simulink model "LCK_0112"  (R2018b)
settings: Solver=FixedStepDiscrete  StartTime=0.0  StopTime=inf  FixedStep=0.01  RelTol=1e-3
PostLoadFcn:
  | if any(exist('dsrtsu_mdlpostloadfcn', 'file') ~= 0), dsrtsu_mdlpostloadfcn('Execute', bdroot); end
values from neighbouring files (symbols this model uses):
  C_DEG2RAD = 0.0175    [LCK_Macro.sldd]
  C_KPH2MPS = 0.2778    [LCK_Macro.sldd]
  C_NEARZERO = 0.0001    [LCK_Macro.sldd]
  C_ONE = 1.0    [LCK_Macro.sldd]
  C_RAD2DEG = 57.2958    [LCK_Macro.sldd]
  C_ZERO = 0.0    [LCK_Macro.sldd]
  k_accel_pedal_pos_per_speed_x : value not decoded    [LCK_LogicPara.sldd]
  k_accel_pedal_pos_per_speed_z : value not decoded    [LCK_LogicPara.sldd]
  k_brake_suprress_hold = 1000.0    [LCK_LogicPara.sldd]
  k_driver_appl_torque_filt = 50.0    [LCK_LogicPara.sldd]
  k_driver_suppression_hold_time = 3000.0    [LCK_LogicPara.sldd]
  k_hands_on_wheel_hold_msec = 500.0    [LCK_LogicPara.sldd]
  k_hands_on_wheel_torque_hi = 0.2    [LCK_LogicPara.sldd]
  k_hands_on_wheel_torque_lo = 0.15    [LCK_LogicPara.sldd]
  k_handsoff_delay_cycles = 50.0    [LCK_LogicPara.sldd]
  k_handsoff_torq_Lo_CR = 0.3    [LCK_LogicPara.sldd]
  k_handson_delay_cycles = 5.0    [LCK_LogicPara.sldd]
  k_HighAccel_suppress_hold = 3000.0    [LCK_LogicPara.sldd]
  k_HLR_suprress_hold = 3000.0    [LCK_LogicPara.sldd]
  k_hs_StrAng_CR_threshold_z : value not decoded    [LCK_LogicPara.sldd]
  k_LC_Exit_Switch = 0.0    [LCK_LogicPara.sldd]
  k_LCG_Configured = 1.0    [LCK_LogicPara.sldd]
  k_LCK_A0_Rdy2Act_UseConst = 0.0    [LCK_LogicPara.sldd]
  k_LCK_A0Fac_ActSta : value not decoded    [LCK_CtrlPara.sldd]
  k_LCK_A0Fac_DrvStm : value not decoded    [LCK_CtrlPara.sldd]
  k_LCK_A0Shift_LftCurv : value not decoded    [LCK_CtrlPara.sldd]
  k_LCK_A0Shift_RgtCurv : value not decoded    [LCK_CtrlPara.sldd]
  k_LCK_A0Shift_StraLan = 0.0    [LCK_CtrlPara.sldd]
  k_LCK_A0ShiftFac_Dy_LftCurv : value not decoded    [LCK_CtrlPara.sldd]
  k_LCK_A0ShiftFac_Dy_RgtCurv : value not decoded    [LCK_CtrlPara.sldd]
  k_LCK_A0ShiftFac_Vspd : value not decoded    [LCK_CtrlPara.sldd]
  k_LCK_accel_inhibit_thold = 35.0    [LCK_LogicPara.sldd]
  k_LCK_Active2Ready_Mask = 255.0    [LCK_LogicPara.sldd]
  k_LCK_CvatRateBks : value not decoded    [LCK_CtrlPara.sldd]
  k_LCK_CvatrBks : value not decoded    [LCK_CtrlPara.sldd]
  k_LCK_DFac_Dy : value not decoded    [LCK_CtrlPara.sldd]
  k_LCK_DFac_Dy_Curv : value not decoded    [LCK_CtrlPara.sldd]
  k_LCK_DFac_HaCurCen : value not decoded    [LCK_CtrlPara.sldd]
  k_LCK_DFac_HaCurSid : value not decoded    [LCK_CtrlPara.sldd]
  k_LCK_DFac_HadCurCen : value not decoded    [LCK_CtrlPara.sldd]
  k_LCK_DFac_HadCurSid : value not decoded    [LCK_CtrlPara.sldd]
  k_LCK_DFac_HadStrCen : value not decoded    [LCK_CtrlPara.sldd]
  k_LCK_DFac_HadStrSid : value not decoded    [LCK_CtrlPara.sldd]
  k_LCK_DFac_HaStrCen : value not decoded    [LCK_CtrlPara.sldd]
  k_LCK_DFac_HaStrSid : value not decoded    [LCK_CtrlPara.sldd]
  k_LCK_DFac_Rad : value not decoded    [LCK_CtrlPara.sldd]
  k_LCK_DFac_SA_CurCen : value not decoded    [LCK_CtrlPara.sldd]
  k_LCK_DFac_SA_CurSid : value not decoded    [LCK_CtrlPara.sldd]
  k_LCK_DFac_SA_StrCen : value not decoded    [LCK_CtrlPara.sldd]
  k_LCK_DFac_SA_StrSid : value not decoded    [LCK_CtrlPara.sldd]
  k_LCK_DFac_SS_CurCen : value not decoded    [LCK_CtrlPara.sldd]
  k_LCK_DFac_SS_CurSid : value not decoded    [LCK_CtrlPara.sldd]
  k_LCK_DFac_SS_StrCen : value not decoded    [LCK_CtrlPara.sldd]
  k_LCK_DFac_SS_StrSid : value not decoded    [LCK_CtrlPara.sldd]
  k_LCK_DFac_Vspd : value not decoded    [LCK_CtrlPara.sldd]
  k_LCK_DlyTm_DrvStim = 0.2    [LCK_CtrlPara.sldd]
  k_LCK_DTermMax = 2.0    [LCK_CtrlPara.sldd]
  k_LCK_DyBks_Curv : value not decoded    [LCK_CtrlPara.sldd]
  k_LCK_Enable_POOnly = 1.0    [LCK_LogicPara.sldd]
  k_LCK_Entry_DistBuffer = 0.1    [LCK_LogicPara.sldd]
  k_LCK_Fac_Vspd2RngThr_FalRec = 0.23    [LCK_CtrlPara.sldd]
  k_LCK_Ffw_CvatSwh = 0.0    [LCK_CtrlPara.sldd]
  k_LCK_Ffw_DyBks : value not decoded    [LCK_CtrlPara.sldd]
  k_LCK_Ffw_TimCon_CmdFlt = 0.0    [LCK_CtrlPara.sldd]
  k_LCK_FfwDeltaFac_Rad_Lft : value not decoded    [LCK_CtrlPara.sldd]
  k_LCK_FfwDeltaFac_Rad_Rgt : value not decoded    [LCK_CtrlPara.sldd]
  k_LCK_FfwDeltaFac_Vspd : value not decoded    [LCK_CtrlPara.sldd]
  k_LCK_FfwFac_CvatRate_Lft : value not decoded    [LCK_CtrlPara.sldd]
  k_LCK_FfwFac_CvatRate_Rgt : value not decoded    [LCK_CtrlPara.sldd]
  k_LCK_FfwFac_Dy : value not decoded    [LCK_CtrlPara.sldd]
  k_LCK_FfwFac_Rad_Lft : value not decoded    [LCK_CtrlPara.sldd]
  k_LCK_FfwFac_Rad_Rgt : value not decoded    [LCK_CtrlPara.sldd]
  k_LCK_FfwFac_Vspd : value not decoded    [LCK_CtrlPara.sldd]
  k_LCK_FfwTorq_Cvat : value not decoded    [LCK_CtrlPara.sldd]
  k_LCK_HAFac_ActSta : value not decoded    [LCK_CtrlPara.sldd]
  k_LCK_HAFac_DrvStm : value not decoded    [LCK_CtrlPara.sldd]
  k_LCK_HaloTime = 2000.0    [LCK_LogicPara.sldd]
  k_LCK_HaloTime_Switch = 0.0    [LCK_LogicPara.sldd]
  k_LCK_HARFac_ActSta : value not decoded    [LCK_CtrlPara.sldd]
  k_LCK_HARFac_DrvStm : value not decoded    [LCK_CtrlPara.sldd]
  k_LCK_Hed_DyBks : value not decoded    [LCK_CtrlPara.sldd]
  k_LCK_HedAngDiffX : value not decoded    [LCK_CtrlPara.sldd]
  k_LCK_HedAngRateDiffX : value not decoded    [LCK_CtrlPara.sldd]
  k_LCK_HndsOnWhel_DlyTm_Idl2Rdy = 0.0    [LCK_LogicPara.sldd]
  k_LCK_host_veh_width = 1.86    [LCK_LogicPara.sldd]
  k_LCK_Idle2Ready_Mask = 239.0    [LCK_LogicPara.sldd]
  k_LCK_Junc_SusTime = 1.0    [LCK_LogicPara.sldd]
  k_LCK_KpKdDecSlopeLmt = 10.0    [LCK_CtrlPara.sldd]
  k_LCK_KpKdIncSlopeLmt = 5.0    [LCK_CtrlPara.sldd]
  k_LCK_Lat_Ctrl_DFac_Lft = 1.0    [LCK_CtrlPara.sldd]
  k_LCK_Lat_Ctrl_DFac_Rgt = 1.05    [LCK_CtrlPara.sldd]
  k_LCK_Lat_Ctrl_Kd = 0.8    [LCK_CtrlPara.sldd]
  k_LCK_Lat_Ctrl_Ki = 0.5    [LCK_CtrlPara.sldd]
  k_LCK_Lat_Ctrl_Kp = 0.7    [LCK_CtrlPara.sldd]
  k_LCK_Lat_Ctrl_Kp_NearGain = 0.7    [LCK_CtrlPara.sldd]
  k_LCK_Lat_Ctrl_PFac_Lft = 1.0    [LCK_CtrlPara.sldd]
  k_LCK_Lat_Ctrl_PFac_Rgt = 1.05    [LCK_CtrlPara.sldd]
  k_LCK_Lat_Ctrl_TimCon_CmdFlt = 5.0    [LCK_CtrlPara.sldd]
  k_LCK_Lat_DFac_Rad : value not decoded    [LCK_CtrlPara.sldd]
  k_LCK_Lat_DFac_SS_Cur : value not decoded    [LCK_CtrlPara.sldd]
  k_LCK_Lat_DFac_SS_Str : value not decoded    [LCK_CtrlPara.sldd]
  k_LCK_Lat_DFac_Vspd : value not decoded    [LCK_CtrlPara.sldd]
  k_LCK_Lat_DyBks : value not decoded    [LCK_CtrlPara.sldd]
  k_LCK_Lat_IFac_Rad : value not decoded    [LCK_CtrlPara.sldd]
  k_LCK_Lat_IFac_Vspd : value not decoded    [LCK_CtrlPara.sldd]
  k_LCK_Lat_ILmtFac_Dy_CurvLan : value not decoded    [LCK_CtrlPara.sldd]
  k_LCK_Lat_ILmtFac_Dy_StraLan : value not decoded    [LCK_CtrlPara.sldd]
  k_LCK_Lat_ILmtFac_Rad : value not decoded    [LCK_CtrlPara.sldd]
  k_LCK_Lat_ILmtFac_Rad_NearGain = 1.0    [LCK_CtrlPara.sldd]
  k_LCK_Lat_ILmtFac_Vspd_CurvLan : value not decoded    [LCK_CtrlPara.sldd]
  k_LCK_Lat_ILmtFac_Vspd_StraLan : value not decoded    [LCK_CtrlPara.sldd]
  k_LCK_Lat_ITermLmt_Dy = 1.0    [LCK_CtrlPara.sldd]
  k_LCK_Lat_KpKdDecSlopeLmt = 10.0    [LCK_CtrlPara.sldd]
  k_LCK_Lat_KpKdIncSlopeLmt = 10.0    [LCK_CtrlPara.sldd]
  k_LCK_Lat_PFac_Dy_InnLftCur : value not decoded    [LCK_CtrlPara.sldd]
  k_LCK_Lat_PFac_Dy_InnRgtCur : value not decoded    [LCK_CtrlPara.sldd]
  k_LCK_Lat_PFac_Dy_OutLftCur : value not decoded    [LCK_CtrlPara.sldd]
  k_LCK_Lat_PFac_Dy_OutRgtCur : value not decoded    [LCK_CtrlPara.sldd]
  k_LCK_Lat_PFac_Dy_Str : value not decoded    [LCK_CtrlPara.sldd]
  k_LCK_Lat_PFac_Rad : value not decoded    [LCK_CtrlPara.sldd]
  ... (+153 more)
undefined symbols (not defined in the file or in its folder): k_LCK_CurvBks, K_LCK_SPA0A1A2_LMRngCmp_y
libraries: LateralControl_fcns_lib x58, simulink x24
(part 2 of 45)

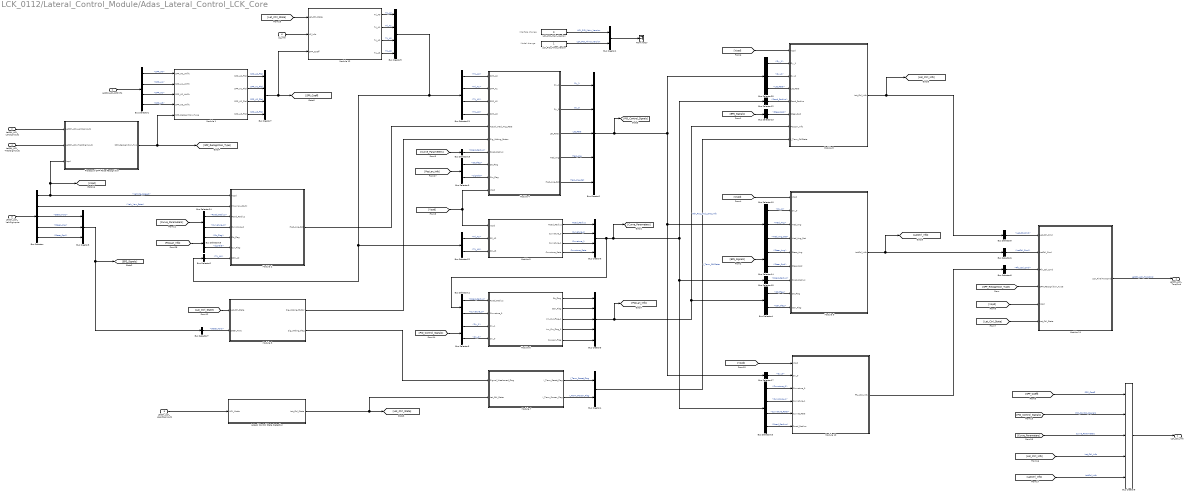
== system LCK_0112/Lateral_Control_Module/Adas_Lateral_Control_LCK_Core ==
  note: Model change
  note: Interface change
  LatCtrl_LCK_SPPInfo : Inport  OutDataTypeStr=Bus: LatCtrl_LCK_SPPInfo_t
  LatCtrl_LCK_LanSigInputs : Inport  Port=2  OutDataTypeStr=Bus: LatCtrl_LCK_LanSigInputs_t
  LatCtrl_LCK_VehSigInputs : Inport  Description=_GWMAB30P4.LCK.000_287_  Port=3  OutDataTypeStr=Bus: LatCtrl_LCK_VehSigInputs_t
  LatCtrl_LCK_TrackSigInputs : Inport  Description=_GWMAB30P4.LCK.000_220_  Port=4  OutDataTypeStr=Bus: LatCtrl_LCK_TrackSigInputs_t
  LatCtrl_LCK_LogicSigInputs : Inport  Description=_GWMAB30P4.LCK.000_293_  Port=5
  LC_Info : Inport  Port=6
  Bus Creator1 : BusCreator  Inputs=2
  Bus Creator2 : BusCreator  Inputs=5
  Bus Creator3 : BusCreator  Inputs=3
  Bus Creator4 : BusCreator  Inputs=2
  Bus Creator5 : BusCreator  Inputs=5
  Bus Creator6 : BusCreator  Inputs=4
  Bus Creator7 : BusCreator  Inputs=4
  Bus Creator8 : BusCreator  Inputs=5
  Bus Creator9 : BusCreator  Inputs=4
  Bus Selector : BusSelector  OutputSignals=Vehicle_Speed,Veh_Yaw_Rate,Steer_Torq,Steer_Ang,Steer_Spd
  Bus Selector1 : BusSelector  OutputSignals=SPP_A0,SPP_A1,SPP_A2,SPP_A3
  Bus Selector10 : BusSelector  OutputSignals=Dy_0,Hed_Ang,Hed_Ang_Rat
  Bus Selector11 : BusSelector  OutputSignals=Road_Radius,Curvature_0
  Bus Selector12 : BusSelector  OutputSignals=Road_Radius
  Bus Selector13 : BusSelector  OutputSignals=Steer_Spd
  Bus Selector14 : BusSelector  OutputSignals=Steer_Ang,Steer_Spd
  Bus Selector15 : BusSelector  OutputSignals=Road_Radius
  Bus Selector16 : BusSelector  OutputSignals=Curvature_0,Curvature_1,Curvature_Rate,Road_Radius
  Bus Selector17 : BusSelector  OutputSignals=Dy_0
  Bus Selector18 : BusSelector  OutputSignals=Str_Flag,signal5
  Bus Selector19 : BusSelector  OutputSignals=Road_Radius
  Bus Selector2 : BusSelector  OutputSignals=Trj_A0
  Bus Selector21 : BusSelector  OutputSignals=Trj_A0,Trj_A1,Trj_A2,Trj_A3
  Bus Selector22 : BusSelector  OutputSignals=Trj_A2,Trj_A3
  Bus Selector24 : BusSelector  OutputSignals=Road_Radius,Curvature_0
  Bus Selector25 : BusSelector  OutputSignals=Dy_1,Dy_0,Lat_Rate
  Bus Selector3 : BusSelector  OutputSignals=Dy_1,Dy_0
  Bus Selector4 : BusSelector  OutputSignals=Str_Flag,Cen_Flag
  Bus Selector5 : BusSelector  OutputSignals=Lat_Ctr_Cmd
  Bus Selector6 : BusSelector  OutputSignals=LatCtrl_Cmd
  Bus Selector7 : BusSelector  OutputSignals=Steer_Torq
  Bus Selector8 : BusSelector  OutputSignals=Ffw_Ctrl_Cmd
  Bus Selector9 : BusSelector  OutputSignals=Str_Flag,signal5
  LCK_PID_Main_Version : Constant  Value=0  OutDataTypeStr=uint8
  LCK_PID_Minor_Version : Constant  OutDataTypeStr=uint8
  Lateral Control State Detection : Subsystem
  Module 1 : Subsystem
  Module 10 : Subsystem
  Module 11 : Subsystem
  Module 12 : Subsystem
  Module 2 : Subsystem
  Module 3 : Subsystem
  Module 4 : Subsystem
  Module 5 : Subsystem
  Module 6 : Subsystem
  Module 7 : Subsystem
  Module 8 : Subsystem
  Module 9 : Subsystem
  Process of SPP False Recognition : Subsystem
  Terminator : Terminator
  LCK_Ctrl_Info : Outport  Description=_GWMAB30P4.LCK.000_318_  OutDataTypeStr=single
  LatCtrl_LCK_TorqCmd : Outport  Description=_GWMAB30P4.LCK.000_318_  Port=2  OutDataTypeStr=single
  wires:
  LCK_PID_Main_Version/1 -> Bus Creator1/1  "LCK_PID_Main_Version"
  Bus Creator7/1 -> Module 12/3(SPP_Coeff), [SPP_Coeff]
  [Vspd] -> Module 4/10(Vspd), Module 5/1(Vspd)
  Bus Selector4/1 -> Module 9/8(Str_Flag)  "<Str_Flag>"
  Bus Selector21/1 -> Module 4/1(SPP_A0)  "<Trj_A0>"
  Lateral Control State Detection/1(Lat_Ctrl_State) -> Module 7/2(Lat_Ctrl_State), [Lat_Ctrl_State]
  [Vspd] -> Module 11/5(Vspd)
  [Curve_Parameters] -> Bus Selector24/1
  Bus Selector16/4 -> Module 10/6(Road_Radius)  "<Road_Radius>"
  Bus Selector7/1 -> Module 3/2(Steer_Torq)  "<Steer_Torq>"
  Module 7/1(I_Term_Reset_Flag) -> Bus Creator4/1  "I_Term_Reset_Flag"
  Bus Selector14/2 -> Module 9/6(Steer_Spd)  "<Steer_Spd>"
  Bus Selector15/1 -> Module 9/7(Road_Radius)  "<Road_Radius>"
  Module 3/2(Sig_Wekng_Flag) -> Module 7/1(Signal_Weakened_Flag)
  Module 1/1(SPP_A0_Fltd) -> Bus Creator7/1  "SPP_A0_Fltd"
  Bus Selector4/2 -> Module 9/9(Cen_Flag)  "<Cen_Flag>"
  Module 2/1(Hed_Ang_Rat) -> Module 4/5(Actual_Hed_Ang_Rate)
  Module 4/1(Dy_1) -> Bus Creator2/1  "Dy_1"
  Bus Selector3/1 -> Module 6/3(Dy_1)  "<Dy_1>"
  Bus Selector1/4 -> Module 1/4(SPP_A3_Unfilt)  "<SPP_A3>"
  [EPS_Signals] -> Bus Selector14/1
  Bus Creator6/1 -> Bus Selector11/1, Bus Selector16/1, Bus Selector15/1, Bus Selector12/1, [Curve_Parameters]
  Module 11/1(LCK_FinalTorqCmd) -> LatCtrl_LCK_TorqCmd/1  "LatCtrl_LCK_TorqCmd"
  Bus Selector12/1 -> Module 8/5(Road_Radius)  "<Road_Radius>"
  Module 6/1(Str_Flag) -> Bus Creator5/1
  Bus Selector25/2 -> Module 8/3(Dy_0)  "<Dy_0>"
  Bus Creator2/1 -> [PID_Control_Signals], Bus Selector25/1, Bus Selector17/1, Bus Selector10/1
  Bus Selector16/1 -> Module 10/3(Curvature_0)  "<Curvature_0>"
  Module 5/2(Curvature_0) -> Bus Creator6/2  "Curvature_0"
  Bus Selector1/2 -> Module 1/2(SPP_A1_Unfilt)  "<SPP_A1>"
  [Vspd] -> Module 8/1(Vspd)
  Process of SPP False Recognition/1(SPP_Recognition_Type) -> [SPP_Recognition_Type], Module 1/5(SPP_Recognition_Type)
  [PosLan_Info] -> Bus Selector9/1
  Bus Selector/1 -> Module 2/1(Vspd), [Vspd], Process of SPP False Recognition/3(Vspd)  "<Vehicle_Speed>"
  Bus Selector1/3 -> Module 1/3(SPP_A2_Unfilt)  "<SPP_A2>"
  Module 5/4(Curvature_Rate) -> Bus Creator6/4  "Curvature_Rate"
  Module 9/1(LatCtrl_Info) -> [LatCtrl_Info], Bus Selector6/1
  Bus Selector/4 -> Bus Creator3/2  "<Steer_Ang>"
  Bus Selector/3 -> Bus Creator3/1  "<Steer_Torq>"
  Bus Selector/5 -> Bus Creator3/3  "<Steer_Spd>"
  Bus Selector21/3 -> Module 4/3(SPP_A2)  "<Trj_A2>"
  LatCtrl_LCK_LanSigInputs/1 -> Process of SPP False Recognition/1(LatCtrl_LCK_LanSigInputs)
  Module 1/2(SPP_A1_Fltd) -> Bus Creator7/2  "SPP_A1_Fltd"
  Bus Creator3/1 -> Bus Selector7/1, [EPS_Signals]
  Module 10/1(Ffw_Ctrl_Info) -> Bus Selector8/1
  [Curve_Parameters] -> Bus Selector19/1
  Module 6/2(Cen_Flag) -> Bus Creator5/2
  LatCtrl_LCK_TrackSigInputs/1 -> Process of SPP False Recognition/2(LatCtrl_LCK_TrackSigInputs)
  Bus Selector2/1 -> Module 2/7(SPP_A0)  "<Trj_A0>"
  Module 7/2(I_Term_Frozen_Flag) -> Bus Creator4/2  "I_Term_Frozen_Flag"
  Bus Selector10/3 -> Module 9/4(Hed_Ang_Rat)  "<Hed_Ang_Rat>"
  Bus Selector18/2 -> Module 2/6(Cur_Flag)  "<signal5>"
  LatCtrl_LCK_LogicSigInputs/1 -> Lateral Control State Detection/1(LCK_Mode)
  Module 1/4(SPP_A3_Fltd) -> Bus Creator7/4  "SPP_A3_Fltd"
  Module 4/5(Hed_Ang_Rat) -> Bus Creator2/5  "Hed_Ang_Rat"
  Bus Selector25/1 -> Module 8/2(Dy_1)  "<Dy_1>"
  Bus Selector11/1 -> Module 6/1(Road_Radius)  "<Road_Radius>"
  Bus Selector22/1 -> Module 5/2(SP_A2)  "<Trj_A2>"
  [Lat_Ctrl_State] -> Module 11/6(Lat_Ctrl_State)
  Bus Selector24/2 -> Module 2/4(Curvature_0)  "<Curvature_0>"
  Module 4/4(Hed_Ang) -> Bus Creator2/4  "Hed_Ang"
  Bus Selector22/2 -> Module 5/3(SP_A3)  "<Trj_A3>"
  [EPS_Signals] -> Bus Selector13/1
  Bus Selector10/1 -> Module 9/2(Dy_0)  "<Dy_0>"
  Bus Selector25/3 -> Module 8/4(Lat_Rate)  "<Lat_Rate>"
  Module 1/3(SPP_A2_Fltd) -> Bus Creator7/3  "SPP_A2_Fltd"
  LatCtrl_LCK_VehSigInputs/1 -> Bus Selector/1
  Bus Creator1/1 -> Terminator/1
  [Lat_Ctrl_State] -> Module 3/1(Lat_Ctrl_State)
  [Vspd] -> Module 9/1(Vspd)
  Bus Selector21/4 -> Module 4/4(SPP_A3)  "<Trj_A3>"
  Bus Selector13/1 -> Module 8/6(Steer_Spd)  "<Steer_Spd>"
  Module 6/4(Inn_Cur_Flag_0) -> Bus Creator5/4
  Module 6/3(Inn_Cur_Flag_1) -> Bus Creator5/3
  Bus Creator5/1 -> Module 8/7(PosLan_Info), Bus Selector4/1, [PosLan_Info]  "Veh_Pos_and_Lane_Info"
  Module 3/1(Sig_Wekng_Factor) -> Module 4/6(Sig_Wekng_Factor)
  Bus Selector16/3 -> Module 10/5(Curvat_Rate)  "<Curvature_Rate>"
  Bus Selector1/1 -> Module 1/1(SPP_A0_Unfilt)  "<SPP_A0>"
  Bus Creator4/1 -> Module 8/8(I_Term_CtrlState)  "I_Term_CtrlState"
  Bus Selector10/2 -> Module 9/3(Hed_Ang)  "<Hed_Ang>"
  Module 4/2(Dy_0) -> Bus Creator2/2  "Dy_0"
  Bus Selector11/2 -> Module 6/2(Curvature_0)  "<Curvature_0>"
  Bus Selector16/2 -> Module 10/4(Curvature_1)  "<Curvature_1>"
  Bus Selector6/1 -> Module 11/2(LatCtrl_Cmd)  "<LatCtrl_Cmd>"
  Bus Selector19/1 -> Module 4/7(Road_Radius)  "<Road_Radius>"
  Bus Selector8/1 -> Module 11/3(Ffw_Ctrl_Cmd)  "<Ffw_Ctrl_Cmd>"
  LCK_PID_Minor_Version/1 -> Bus Creator1/2  "LCK_PID_Minor_Version"
  Module 8/1(Lat_Ctrl_Info) -> [Lat_Ctrl_Info], Bus Selector5/1
  Bus Selector3/2 -> Module 6/4(Dy_0)  "<Dy_0>"
  [Vspd] -> Module 10/1(Vspd)
  Module 5/3(Curvature_1) -> Bus Creator6/3  "Curvature_1"
  Bus Selector9/2 -> Module 4/9(Cur_Flag)  "<signal5>"
  [PID_Control_Signals] -> Bus Selector3/1
  Bus Selector18/1 -> Module 2/5(Str_Flag)  "<Str_Flag>"
  Bus Selector9/1 -> Module 4/8(Str_Flag)  "<Str_Flag>"
  Bus Selector21/2 -> Module 4/2(SPP_A1)  "<Trj_A1>"
  [SPP_Recognition_Type] -> Module 11/4(SPP_Recognition_Type)
  [PosLan_Info] -> Bus Selector18/1
  Bus Selector14/1 -> Module 9/5(Steer_Ang)  "<Steer_Ang>"
  Module 5/1(Road_Radius) -> Bus Creator6/1  "Road_Radius"
  Module 4/3(Lat_Rate) -> Bus Creator2/3  "Lat_Rate"
  Module 6/5(Cur_Lan_Flag) -> Bus Creator5/5
  LatCtrl_LCK_SPPInfo/1 -> Bus Selector1/1
  Bus Selector17/1 -> Module 10/2(Dy_0)  "<Dy_0>"
  Bus Selector/2 -> Module 2/2(IMU_Yaw_Rt_Pri)  "<Veh_Yaw_Rate>"
  Bus Selector24/1 -> Module 2/3(Road_Radius)  "<Road_Radius>"
  [SPP_Coeff] -> Bus Creator8/1  "SPP_Coeff"
  [PID_Control_Signals] -> Bus Creator8/2  "PID_Control_Signals"
  [Curve_Parameters] -> Bus Creator8/3  "Curve_Parameters"
  Bus Selector5/1 -> Module 11/1(Lat_Ctrl_Cmd)  "<Lat_Ctr_Cmd>"
  [Lat_Ctrl_Info] -> Bus Creator8/4  "Lat_Ctrl_Info"
  [LatCtrl_Info] -> Bus Creator8/5  "LatCtrl_Info"
  Bus Creator8/1 -> LCK_Ctrl_Info/1
  LC_Info/1 -> Module 12/2(LC_Info)
  Module 12/1(Trj_A0) -> Bus Creator9/1  "Trj_A0"
  Module 12/2(Trj_A1) -> Bus Creator9/2  "Trj_A1"
  Module 12/3(Trj_A2) -> Bus Creator9/3  "Trj_A2"
  Module 12/4(Trj_A3) -> Bus Creator9/4  "Trj_A3"
  Bus Creator9/1 -> Bus Selector21/1, Bus Selector22/1, Bus Selector2/1
  [Lat_Ctrl_State] -> Module 12/1(Lat_Ctrl_State)
